simulink model "pinpt_decomposer"  (Simulink 7.9)
settings: Solver=ode45  StartTime=0.0  StopTime=10.0  RelTol=1e-3
settings Model: Creator=Scott  LastModifiedBy=Scott

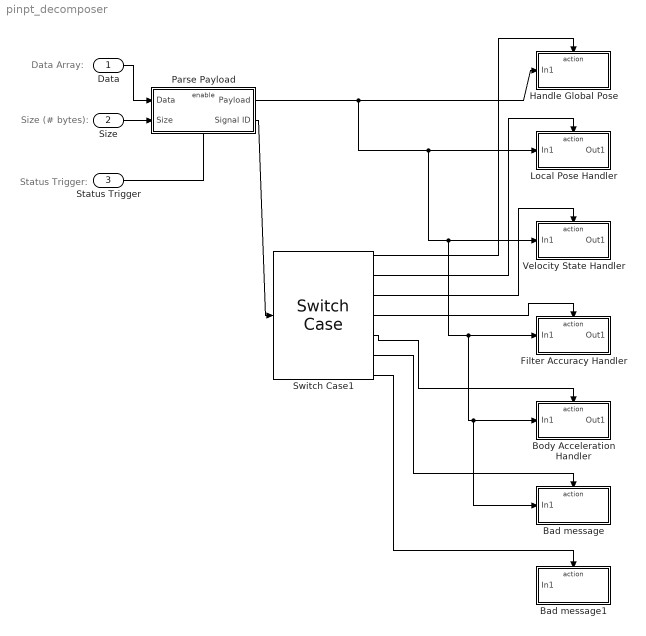
== system pinpt_decomposer ==
  note: Data Array:
  note: Size (# bytes):
  note: Status Trigger:
  Data : Inport  OutDataTypeStr=uint32  Interpolate=off
  Size : Inport  Port=2  OutDataTypeStr=int32
  Status Trigger : Inport  Port=3  OutDataTypeStr=boolean
  Bad message : Subsystem  TreatAsAtomicUnit=on
  Bad message1 : Subsystem  TreatAsAtomicUnit=on
  Body Acceleration Handler : Subsystem  TreatAsAtomicUnit=on
  Filter Accuracy Handler : Subsystem  TreatAsAtomicUnit=on
  Handle Global Pose : Subsystem  TreatAsAtomicUnit=on
  Local Pose Handler : Subsystem  TreatAsAtomicUnit=on
  Parse Payload : Subsystem  TreatAsAtomicUnit=on
  Switch Case1 : SwitchCase  CaseConditions={6, 7, 8, 10, 12, -1}
  Velocity State Handler : Subsystem  TreatAsAtomicUnit=on
  wires:
  Status Trigger/1 -> Parse Payload/Enable
  Size/1 -> Parse Payload/2(Size)
  Data/1 -> Parse Payload/1(Data)
  Parse Payload/2(Signal ID) -> Switch Case1/1
  Switch Case1/5 -> Body Acceleration Handler/Action
  Switch Case1/4 -> Filter Accuracy Handler/Action
  Switch Case1/3 -> Velocity State Handler/Action
  Switch Case1/2 -> Local Pose Handler/Action
  Switch Case1/1 -> Handle Global Pose/Action
  Parse Payload/1(Payload) -> Handle Global Pose/1(In1), Local Pose Handler/1(In1), Velocity State Handler/1(In1), Filter Accuracy Handler/1(In1), Body Acceleration Handler/1(In1), Bad message/1(In1)
  Switch Case1/6 -> Bad message/Action
  Switch Case1/7 -> Bad message1/Action

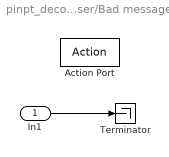
== system pinpt_decomposer/Bad message ==
  In1 : Inport
  Action Port : ActionPort  ActionType=case
  Terminator : Terminator
  wires:
  In1/1 -> Terminator/1

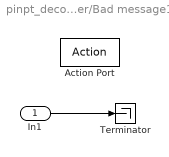
== system pinpt_decomposer/Bad message1 ==
  In1 : Inport
  Action Port : ActionPort  ActionType=default
  Terminator : Terminator
  wires:
  In1/1 -> Terminator/1

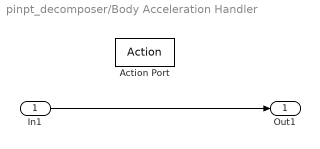
== system pinpt_decomposer/Body Acceleration Handler ==
  In1 : Inport
  Action Port : ActionPort  ActionType=case
  Out1 : Outport
  wires:
  In1/1 -> Out1/1

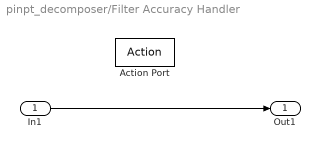
== system pinpt_decomposer/Filter Accuracy Handler ==
  In1 : Inport
  Action Port : ActionPort  ActionType=case
  Out1 : Outport
  wires:
  In1/1 -> Out1/1

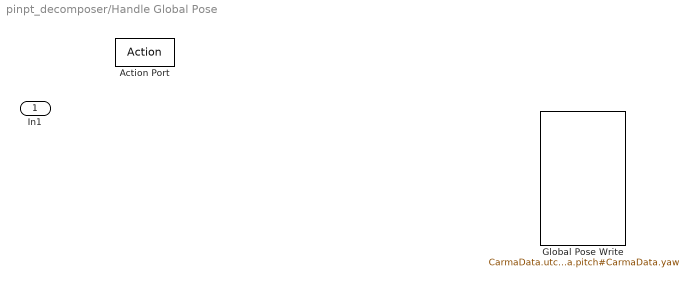
== system pinpt_decomposer/Handle Global Pose ==
  In1 : Inport
  Action Port : ActionPort  ActionType=case
  Global Pose Write : DataStoreWrite  DataStoreName=CarmaData  DataStoreElements=CarmaData.utc_time_s#CarmaData.latitude#CarmaData.longitude#CarmaData.altitude#CarmaData.roll#CarmaData.pitch#CarmaData.yaw

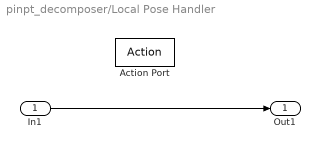
== system pinpt_decomposer/Local Pose Handler ==
  In1 : Inport
  Action Port : ActionPort  ActionType=case
  Out1 : Outport
  wires:
  In1/1 -> Out1/1

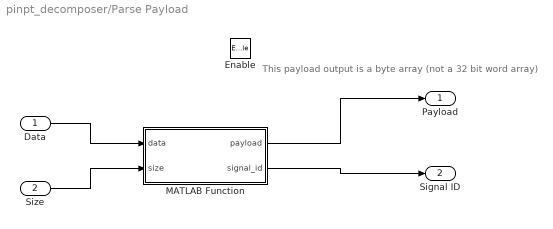
== system pinpt_decomposer/Parse Payload ==
  note: This payload output is a byte array
      | (not a 32 bit word array)
  Data : Inport  OutDataTypeStr=uint32
  Size : Inport  Port=2  OutDataTypeStr=int32
  Enable : EnablePort
  MATLAB Function : MATLAB Function  TreatAsAtomicUnit=on
  Payload : Outport  OutDataTypeStr=uint8
  Signal ID : Outport  Port=2  OutDataTypeStr=uint8
  wires:
  Data/1 -> MATLAB Function/1(data)
  Size/1 -> MATLAB Function/2(size)
  MATLAB Function/1(payload) -> Payload/1
  MATLAB Function/2(signal_id) -> Signal ID/1

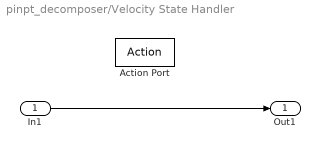
== system pinpt_decomposer/Velocity State Handler ==
  In1 : Inport
  Action Port : ActionPort  ActionType=case
  Out1 : Outport
  wires:
  In1/1 -> Out1/1

== matlab function Parse Payload/MATLAB Function ==
  data: payload output double; signal_id output double; data input double; size input double
% IN:
% data - array of unsigned integers (32 bits) containing UDP packet data
% size - signed 32 bit integer representing the number of bytes in the UDP
%        packet
%
% OUT:
% payload - array of 8-bit unsigned integers contiaining the payload of the
%           message
% type    - 8-bit unsigned integer representing the message ID of the
%           payload data (each pinpoint message has a unique id)

function [payload, signal_id]= parseSignal(data, size)
%#codegen

%Constants
HEADER_SIZE = 2;
MSGTYPE_SIGNAL_EMITTED = 3;


% Make sure there's enough data for the header
if size < HEADER_SIZE
    signal_id = uint8(-1);
    payload = uint8(0);
    return
end
controlbyte = bitand(data(1), 255); % pull out the first byte
signal_id = uint8(bitshift(bitand(data(1), 65280), -8)); % pull out second byte

% check for (and ignore) a protocol message
if bitand(controlbyte, 128) > 0 %bit 7
    signal_id = uint8(-1);
    payload = uint8(0);
    return
end

% Ignore anything that's not a signal emitted message
if bitshift(bitand(controlbyte, 120), -3) ~= MSGTYPE_SIGNAL_EMITTED %bits 6:3
    signal_id = uint8(-1);
    payload = uint8(0);
    return
end

size_enum = bitand(controlbyte, 3); % 0: no data, 1: single byte size, 2: 2 two byte size, 3: 4 byte size

payload_size = 0;
payload_start = 3;

if size_enum == 1
    payload_size = bitshift(bitand(data(1), 16711680), -16); %third byte
    payload_start = payload_start + 1;
elseif size_enum == 2
    payload_size = bitshift(bitand(data(1), 4294901760), -16); %third and fourth bytes
    payload_start = payload_start + 2;
elseif size_enum == 3
    payload_size = bitshift(bitand(data(1), 4294901760), -16); %third and fourth bytes
    payload_size = bitor(payload_size, bitshift(bitand(data(2), 65535), 16)); %first & second bytes of second integer
    payload_start = payload_start + 4;
end

% make sure there's enough data to fill in the payload
if payload_size > (size - HEADER_SIZE)
    signal_id = uint8(-1);
    payload = uint8(0);
    return
end

% payload = zeros(payload_size, 'uint8');
% num_words = payload_size / 4;

payload = uint8(wordsToBytes(data, payload_size, payload_start));
    
end

% convert an array of 32 bit words to an array of 8-bit bytes.
function [byte_array] = wordsToBytes(word_array, num_bytes, byte_offset)

byte_array = zeros(num_bytes, 'uint8');
current_word = 1;

% handle initial byte offset
while byte_offset >= 4
    current_word = current_word + 1;
    byte_offset = byte_offset - 4;
end

input_byte = byte_offset;
output_byte = 1;

for i=current_byte:num_bytes
    byte_array(output_byte) = bitand(bitshift(word_array(current_word), mod(input_byte, 4)*8), 255);
    input_byte = input_byte + 1;
    output_byte = output_byte + 1;
end

end
